simulink model "sp1"  (R2020b)
settings: Solver=VariableStepAuto  StartTime=0.0  StopTime=2  RelTol=1e-3
libraries: dspsigops x1
settings Model: Creator=seojoon  LastModifiedBy=seojoon
settings DataIOCC: ReturnWorkspaceOutputs=off

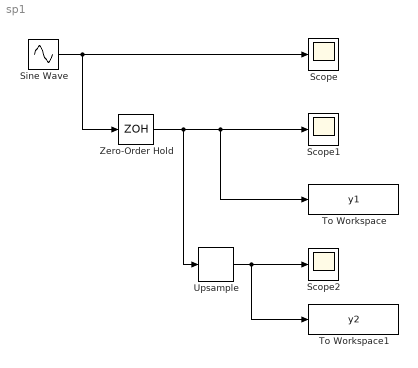
== system sp1 ==
  Scope : Scope
  Scope1 : Scope
  Scope2 : Scope
  Sine Wave : Sin  Amplitude=10  Frequency=2*pi*1  SampleTime=0
  To Workspace : ToWorkspace  VariableName=y1  SaveFormat=Structure With Time  SampleTime=-1
  To Workspace1 : ToWorkspace  VariableName=y2  SaveFormat=Structure With Time  SampleTime=-1
  Upsample : dspsigops/Upsample  N=2  phase=0  RateOptions=Allow multirate processing  ic=0  mode=Unused parameter value
  Zero-Order Hold : ZeroOrderHold  SampleTime=1/20
  wires:
  Sine Wave/1 -> Zero-Order Hold/1, Scope/1
  Zero-Order Hold/1 -> Upsample/1, To Workspace/1, Scope1/1
  Upsample/1 -> Scope2/1, To Workspace1/1
